simulink model "Lab_Simulink"  (R2014b)
settings: Solver=ode45  StartTime=0.0  StopTime=1000  RelTol=1e-3
settings Model: Creator=Пользователь  LastModifiedBy=Пользователь

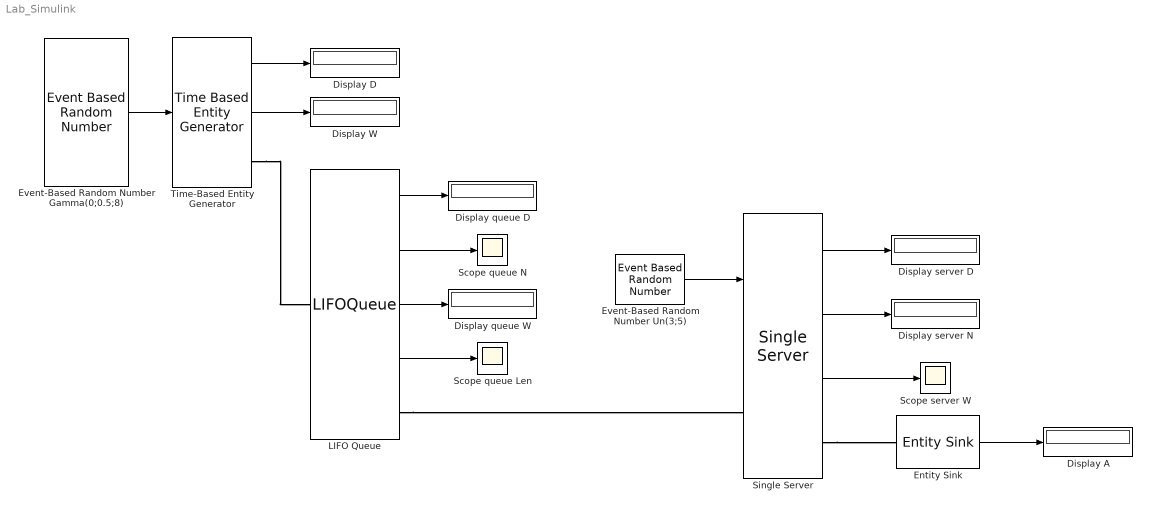
== system Lab_Simulink ==
  Display A : Display
  Display D : Display
  Display W : Display
  Display queue D : Display
  Display queue W : Display
  Display server D : Display
  Display server N : Display
  Entity Sink : EntitySink  StatNumberArrived=on
  Event-Based Random Number Gamma(0;0.5;8) : EventBasedRandomNumber  Distribution=Gamma  scaleGam=0.5  shapeGam=8
  Event-Based Random Number Un(3;5) : EventBasedRandomNumber  Distribution=Uniform  minUnif=3  maxUnif=5  Seed=54321
  LIFO Queue : LIFOQueue  Capacity=3  StatNumberDeparted=on  StatNumberInBlock=on  StatAverageWait=on  StatAverageQueueLength=on
      settings: OutputPortMap=o0,o1,o2,o3
  Scope queue Len : Scope
      settings: SaveName=Lenqueue  MaxDataPoints=50000
  Scope queue N : Scope
      settings: SaveName=Nqueue  MaxDataPoints=50000
  Scope server W : Scope
      settings: SaveName=Wserver  MaxDataPoints=50000
  Single Server : SingleServer  ServiceTimeFrom=Signal port t  StatNumberDeparted=on  StatNumberInBlock=on  StatAverageWait=on
      settings: OutputPortMap=o0,o1,o4
  Time-Based Entity Generator : TimeBasedEntityGenerator  GenerateEntitiesUpon=Intergeneration time from port t  StatNumberDeparted=on  StatAverageIntergenerationTime=on
      settings: OutputPortMap=o0,o2
  wires:
  Event-Based Random Number Gamma(0;0.5;8)/1 -> Time-Based Entity Generator/1
  Time-Based Entity Generator/1 -> Display D/1
  Time-Based Entity Generator/2 -> Display W/1
  LIFO Queue/1 -> Display queue D/1
  LIFO Queue/2 -> Scope queue N/1
  LIFO Queue/3 -> Display queue W/1
  LIFO Queue/4 -> Scope queue Len/1
  Single Server/3 -> Scope server W/1
  Single Server/2 -> Display server N/1
  Single Server/1 -> Display server D/1
  Event-Based Random Number Un(3;5)/1 -> Single Server/1
  Entity Sink/1 -> Display A/1
  connections:
  Time-Based Entity Generator/RConn1 -- LIFO Queue/LConn1
  LIFO Queue/RConn1 -- Single Server/LConn1
  Single Server/RConn1 -- Entity Sink/LConn1
